simulink model "simulink_3_1f"  (R2025b)
settings: Solver=VariableStepAuto  StartTime=0.0  StopTime=5  RelTol=1e-3
settings Model: Creator=getrj  LastModifiedBy=owenm
settings SolverCC: ZeroCrossAlgorithm=Adaptive
settings DebuggingCC: IgnoredZcDiagnostic=none

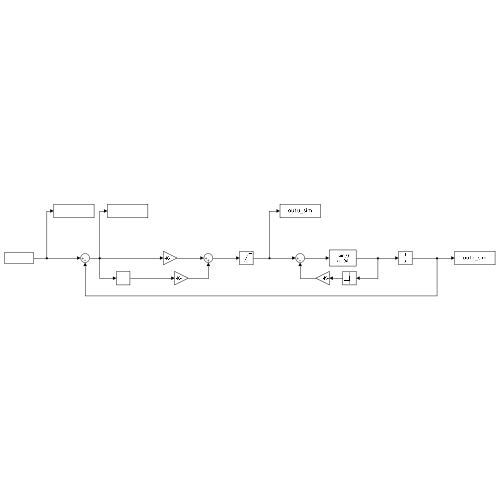
[thumbnail: Simulink's stored preview of the top-level diagram]
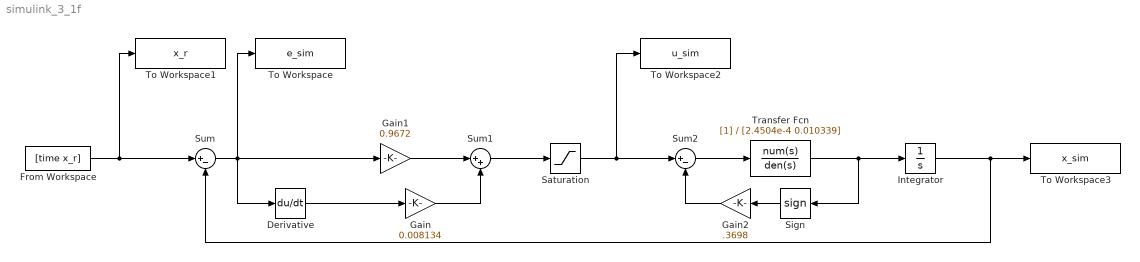
== system simulink_3_1f ==
  Derivative : Derivative
  From Workspace : FromWorkspace  VariableName=[time x_r]
  Gain : Gain  Gain=0.008134
  Gain1 : Gain  Gain=0.9672
  Gain2 : Gain  Gain=.3698
  Integrator : Integrator
  Saturation : Saturate  UpperLimit=10  LowerLimit=-10
  Sign : Signum
  Sum : Sum  Inputs=|+-
  Sum1 : Sum  Inputs=|++
  Sum2 : Sum  Inputs=|+-
  To Workspace : ToWorkspace  VariableName=e_sim  SaveFormat=Timeseries  SampleTime=-1
  To Workspace1 : ToWorkspace  VariableName=x_r  SaveFormat=Timeseries  SampleTime=-1
  To Workspace2 : ToWorkspace  VariableName=u_sim  SaveFormat=Timeseries  SampleTime=-1
  To Workspace3 : ToWorkspace  VariableName=x_sim  SaveFormat=Timeseries  SampleTime=-1
  Transfer Fcn : TransferFcn  Denominator=[2.4504e-4 0.010339]
  wires:
  From Workspace/1 -> To Workspace1/1, Sum/1
  Sum/1 -> To Workspace/1, Derivative/1, Gain1/1
  Gain1/1 -> Sum1/1
  Gain/1 -> Sum1/2
  Sum1/1 -> Saturation/1
  Saturation/1 -> Sum2/1, To Workspace2/1
  Integrator/1 -> To Workspace3/1, Sum/2
  Derivative/1 -> Gain/1
  Transfer Fcn/1 -> Sign/1, Integrator/1
  Sum2/1 -> Transfer Fcn/1
  Gain2/1 -> Sum2/2
  Sign/1 -> Gain2/1
